simulink model "quadrotorVehicle_baseline_workshop"  (R2023b)
settings: Solver=VariableStepAuto  StartTime=0.0  StopTime=600  MaxStep=0.1  RelTol=1e-3  EnableMultiTasking=on
InitFcn:
  | % load parameters of the default quadrotor
  | disp('Quadrotor parameters loaded by InitFcn')
  | mdl_quadrotor;
  | waypoints = randi([-500,500],10,2);
libraries: simulink x2, slpidlib x1, roblocks x1
settings Model: PacingRate=10  Creator=corkep  LastModifiedBy=mejiasal
settings SolverCC: AlgebraicLoopSolver=TrustRegion
settings DataIOCC: LimitDataPoints=on  SaveFormat=Array  ReturnWorkspaceOutputs=off
settings OptimizationCC: BlockReduction=off  BooleanDataType=off  ReuseModelBlockBuffer=off  LifeSpan=inf
settings DebuggingCC: SaveWithParameterizedLinksMsg=none  MergeDetectMultiDrivingBlocksExec=none  SignalResolutionControl=TryResolveAllWithWarning  UnconnectedInputMsg=warning  UnconnectedOutputMsg=warning  UnconnectedLineMsg=warning  SFUnexpectedBacktrackingDiag=warning  SFNoUnconditionalDefaultTransitionDiag=warning  SFExecutionAtInitializationDiag=none  ArithmeticOperatorsInVariantConditions=warning
settings HardwareCC: ProdBitPerPointer=32  ProdBitPerSizeT=32  ProdBitPerPtrDiffT=32  ProdLargestAtomicFloat=None  ProdIntDivRoundTo=Undefined  ProdEndianess=Unspecified  ProdWordSize=32  ProdHWDeviceType=32-bit Generic  TargetUnknown=on
settings ModelReferenceCC: EnableRefExpFcnMdlSchedulingChecks=on  PropagateSignalLabelsOutOfModel=off
settings SFSimCC: SimUseLocalCustomCode=off  CustomCodeUndefinedFunction=UseInterfaceOnly
settings RTWCC: RTWUseLocalCustomCode=off
settings CodeAppCC: StateflowObjectComments=on
settings GRTTargetCC: TargetLangStandard=C89/C90 (ANSI)
settings ConfigComp: CovMetricSettings=dw  CovSaveCumulativeToWorkspaceVar=on  CovSaveSingleToWorkspaceVar=on  CovExternalEMLEnable=off  CovSFcnEnable=off

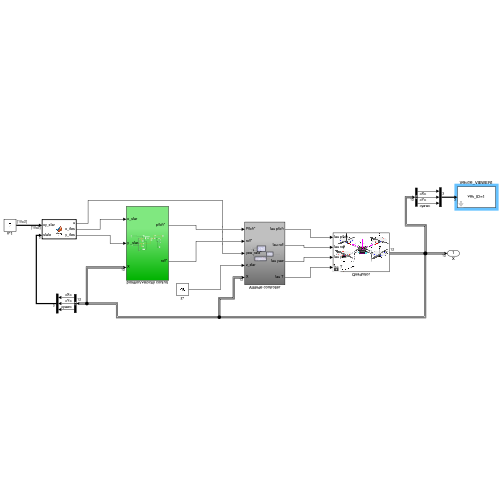
[thumbnail: Simulink's stored preview of the top-level diagram]
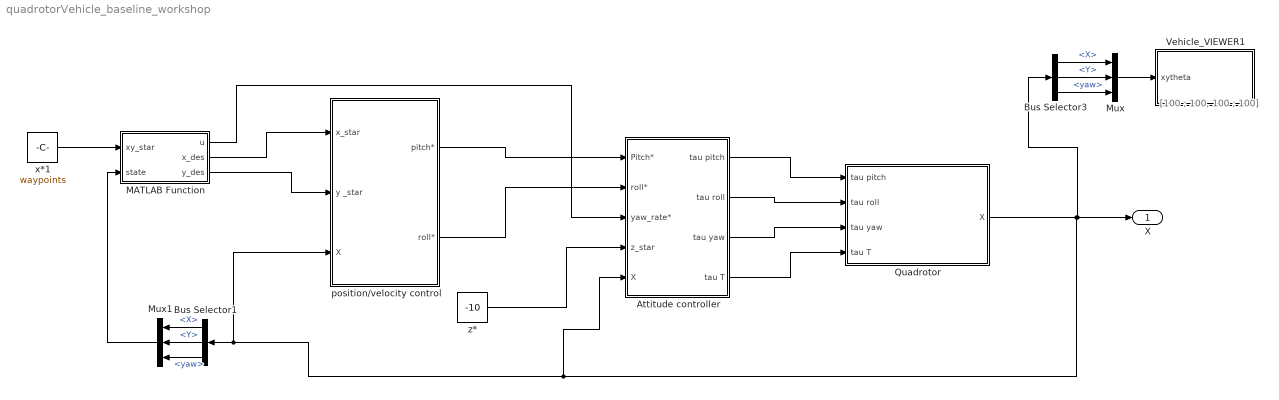
== system quadrotorVehicle_baseline_workshop ==
  note: [100 ; 100, 100 ; 100]
  Attitude controller : Subsystem
  Bus Selector1 : BusSelector  OutputSignals=X,Y,yaw
  Bus Selector3 : BusSelector  OutputSignals=X,Y,yaw
  MATLAB Function : MATLAB Function  TreatAsAtomicUnit=on
  Mux : Mux  Inputs=3
  Mux1 : Mux  Inputs=3
  Quadrotor : Subsystem
      mask Display: image('quadrotor.png');
  Vehicle_VIEWER1 : Subsystem  mask{wp_mat=waypoints, veh_ID_num=1, veh_init_xytheta=[0 0 0], Ts=5}
      mask prompts: wp_mat "Waypoint matrix for arena [x_col, y_col, z_col, angle_col] (m, deg)"; veh_ID_num "Vehicle ID number"; veh_init_xytheta "Initial pose [x,y, psi]"; Ts "Sample time for updating animation (secs)"
      mask TypeOptions veh_ID_num: 1 | 2 | 3 | 4
      mask DialogControl Control2 Prompt: Animate simulation of Robot
      mask Display: fprintf('veh_ID=%d',veh_ID_num);
  position/velocity control : Subsystem
  x*1 : Constant  Value=waypoints
  z* : Constant  Value=-10
  X : Outport
  wires:
  Bus Selector3/1 -> Mux/1  "<X>"
  Bus Selector3/2 -> Mux/2  "<Y>"
  Bus Selector3/3 -> Mux/3  "<yaw>"
  Mux/1 -> Vehicle_VIEWER1/1(xytheta)
  position/velocity control/2(roll*) -> Attitude controller/2(roll*)
  z*/1 -> Attitude controller/4(z_star)
  position/velocity control/1("pitch*  ") -> Attitude controller/1(Pitch*)
  Attitude controller/1(tau pitch) -> Quadrotor/1(tau pitch)
  Attitude controller/2(tau roll) -> Quadrotor/2(tau roll)
  Attitude controller/3(tau yaw) -> Quadrotor/3(tau yaw)
  Attitude controller/4(tau T) -> Quadrotor/4(tau T)
  Quadrotor/1(X) -> Bus Selector3/1, X/1, Attitude controller/5(X), position/velocity control/3(X), Bus Selector1/1
  Bus Selector1/1 -> Mux1/1  "<X>"
  Bus Selector1/2 -> Mux1/2  "<Y>"
  Bus Selector1/3 -> Mux1/3  "<yaw>"
  Mux1/1 -> MATLAB Function/2(state)
  MATLAB Function/1(u) -> Attitude controller/3(yaw_rate*)
  MATLAB Function/2(x_des) -> position/velocity control/1(x_star)
  MATLAB Function/3(y_des) -> position/velocity control/2(y _star)
  x*1/1 -> MATLAB Function/1(xy_star)

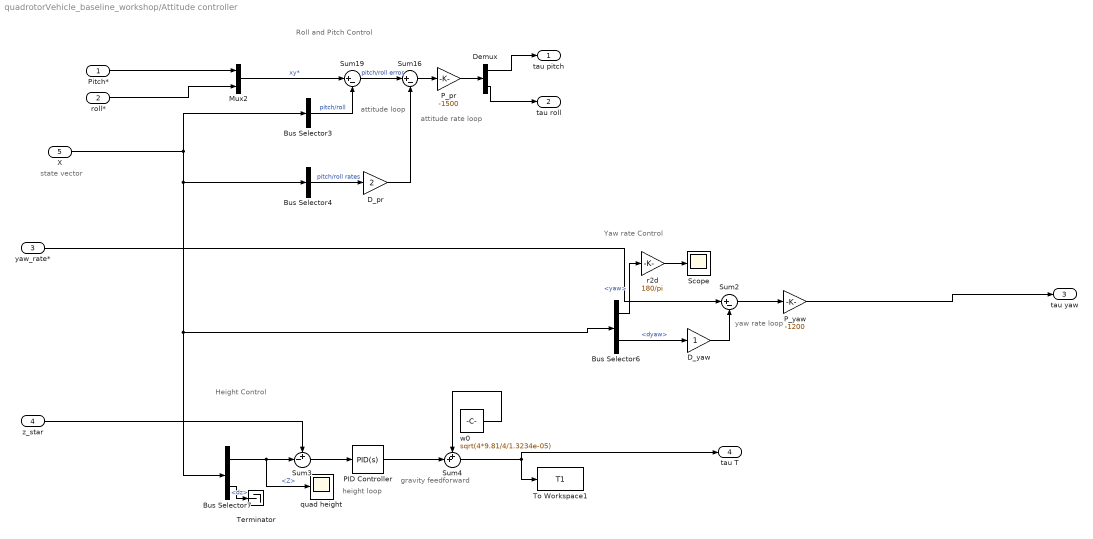
== system quadrotorVehicle_baseline_workshop/Attitude controller ==
  note: Height Control
  note: Yaw rate Control
  note: Roll and Pitch Control
  note: state vector
  note: gravity feedforward
  note: attitude rate
      | loop
  note: height
      | loop
  note: attitude
      | loop
  note: yaw rate
      | loop
  Pitch* : Inport
  roll* : Inport  Port=2
  yaw_rate* : Inport  Port=3
  z_star : Inport  Port=4
  X : Inport  Port=5
  Bus Selector3 : BusSelector  OutputSignals=pitch,roll  OutputAsBus=on
  Bus Selector4 : BusSelector  OutputSignals=dpitch,droll  OutputAsBus=on
  Bus Selector6 : BusSelector  OutputSignals=yaw,dyaw
  Bus Selector7 : BusSelector  OutputSignals=Z,dz
  D_pr : Gain  Gain=2
  D_yaw : Gain
  Demux : Demux  Outputs=2
  Mux2 : Mux  Inputs=2
  PID Controller : slpidlib/PID Controller  Controller=PID  Form=Parallel  TimeDomain=Continuous-time  UseExternalTs=off  SampleTime=-1  IntegratorMethod=Forward Euler  FilterMethod=Forward Euler  ControllerParametersSource=internal  P=-7.01788852939257  I=-0.1  UseKiTs=off  D=-38  N=5.45397025421619  UseFilter=on  TunerSelectOption=Transfer Function Based (PID Tuner App)  InitialConditionSource=internal  InitialConditionForIntegrator=0  InitialConditionForFilter=0  DifferentiatorICPrevScaledInput=0  ExternalReset=none  TrackingMode=off  Kt=1  LimitOutput=off  SatLimitsSource=internal  UpperSaturationLimit=inf  LowerSaturationLimit=-inf  LinearizeAsGain=on  AntiWindupMode=none  Kb=1  LimitIntegrator=off  UpperIntegratorSaturationLimit=inf  LowerIntegratorSaturationLimit=-inf  POutMin=[]  POutMax=[]  IOutMin=[]  IOutMax=[]  DOutMin=[]  DOutMax=[]  NOutMin=[]  NOutMax=[]  SumOutMin=[]  SumOutMax=[]  SaturationOutMin=[]  SaturationOutMax=[]  PParamMin=[]  PParamMax=[]  IParamMin=[]  IParamMax=[]  DParamMin=[]  DParamMax=[]  NParamMin=[]  NParamMax=[]  KbParamMin=[]  KbParamMax=[]  KtParamMin=[]  KtParamMax=[]  KbOutMin=[]  KbOutMax=[]  KtOutMin=[]  KtOutMax=[]  IntegratorOutMin=[]  IntegratorOutMax=[]  FilterOutMin=[]  FilterOutMax=[]  SumI1OutMin=[]  SumI1OutMax=[]  SumI2OutMin=[]  SumI2OutMax=[]  SumI3OutMin=[]  SumI3OutMax=[]  SumI4OutMin=[]  SumI4OutMax=[]  SumDOutMin=[]  SumDOutMax=[]  DifferentiatorOutMin=[]  DifferentiatorOutMax=[]  FilterDiffOutCoefMin=[]  FilterDiffOutCoefMax=[]  ReciprocalOutMin=[]  ReciprocalOutMax=[]  SumDenOutMin=[]  SumDenOutMax=[]  SumNumOutMin=[]  SumNumOutMax=[]  DivideOutMin=[]  DivideOutMax=[]  UdiffTsProdOutMin=[]  UdiffTsProdOutMax=[]  NTsProdOutMin=[]  NTsProdOutMax=[]  UintegralTsProdOutMin=[]  UintegralTsProdOutMax=[]  UngainTsProdOutMin=[]  UngainTsProdOutMax=[]  ClampingZeroOutDataTypeStr=Inherit: Inherit via back propagation  ClampingZeroOutMin=[]  ClampingZeroOutMax=[]  FilterDenConstantOutDataTypeStr=Inherit: Inherit via back propagation  FilterDenConstantOutMin=[]  FilterDenConstantOutMax=[]  PCopyOutDataTypeStr=Inherit: Inherit via back propagation  PCopyOutMin=[]  PCopyOutMax=[]  NCopyOutDataTypeStr=Inherit: Inherit via back propagation  NCopyOutMin=[]  NCopyOutMax=[]  IntegratorContinuousStateAttributes=''  IntegratorStateMustResolveToSignalObject=off  IntegratorRTWStateStorageClass=Auto  FilterContinuousStateAttributes=''  FilterStateMustResolveToSignalObject=off  FilterRTWStateStorageClass=Auto  ParallelPVariant=InternalParameters  IdealPVariant=Disabled  IVariant=InternalParameters  DVariant=InternalParameters  IntegratorVariant=Continuous  SatVariant=Disabled  AWVariant=Passthrough  PCopyVariant=Disabled  TRVariant=Disabled  FdbkBlocksVariant=Forward  IdealPFdbkVariant=Disabled  SatFdbkVariant=Disabled  DerivativeFilterVariant=ContFilter  NVariant=InternalParameters  NCopyVariant=Disabled  FilterICVariant=InternalICsFilter  IntegratorICVariant=InternalICs  ExternalResetVariant=Disabled  TRSumVariant=Passthrough  SumFdbkVariant=Disabled  SumVariant=Sum_PID  TsampFilterVariant=InternalTs  TsampNgainVariant=Passthrough  TsampIntegralVariant=Disabled_SignalSpec  ExternalSaturationOutDataTypeStr=Inherit: Same as second input
  P_pr : Gain  Gain=-1500
  P_yaw : Gain  Gain=-1200
  Scope : Scope
  Sum16 : Sum  Inputs=|+-
  Sum19 : Sum  Inputs=|+-
  Sum2 : Sum  Inputs=|+-
  Sum3 : Sum  Inputs=+-|
  Sum4 : Sum  Inputs=++|
  Terminator : Terminator
  To Workspace1 : ToWorkspace  VariableName=T1  SampleTime=-1
  quad height : Scope
  r2d : Gain  Gain=180/pi
  w0 : Constant  Value=sqrt(4*9.81/4/1.3234e-05)  SampleTime=0
  tau pitch : Outport  VectorParamsAs1DForOutWhenUnconnected=off
  tau roll : Outport  Port=2  VectorParamsAs1DForOutWhenUnconnected=off
  tau yaw : Outport  Port=3  VectorParamsAs1DForOutWhenUnconnected=off
  tau T : Outport  Port=4  VectorParamsAs1DForOutWhenUnconnected=off
  wires:
  P_pr/1 -> Demux/1
  Demux/1 -> tau pitch/1
  yaw_rate*/1 -> Sum2/1
  roll*/1 -> Mux2/2
  Bus Selector6/1 -> r2d/1  "<yaw>"
  Bus Selector3/1 -> Sum19/2  "pitch/roll"
  PID Controller/1 -> Sum4/2
  Demux/2 -> tau roll/1
  Sum16/1 -> P_pr/1
  Mux2/1 -> Sum19/1  "xy*"
  r2d/1 -> Scope/1
  z_star/1 -> Sum3/1
  Sum19/1 -> Sum16/1  "pitch/roll error"
  Pitch*/1 -> Mux2/1
  D_yaw/1 -> Sum2/2
  Bus Selector6/2 -> D_yaw/1  "<dyaw>"
  Bus Selector4/1 -> D_pr/1  "pitch/roll rates"
  Bus Selector7/1 -> quad height/1, Sum3/2  "<Z>"
  X/1 -> Bus Selector7/1, Bus Selector6/1, Bus Selector4/1, Bus Selector3/1
  Sum2/1 -> P_yaw/1
  Sum3/1 -> PID Controller/1
  w0/1 -> Sum4/1
  D_pr/1 -> Sum16/2
  P_yaw/1 -> tau yaw/1
  Sum4/1 -> tau T/1, To Workspace1/1
  Bus Selector7/2 -> Terminator/1  "<dz>"

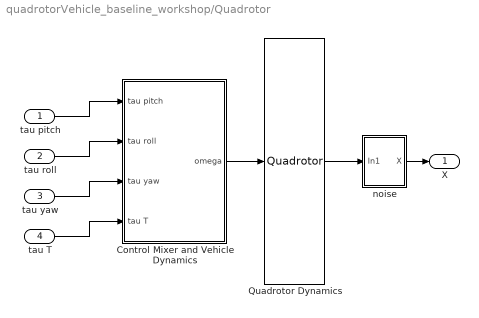
== system quadrotorVehicle_baseline_workshop/Quadrotor ==
  tau pitch : Inport
  tau roll : Inport  Port=2
  tau yaw : Inport  Port=3
  tau T : Inport  Port=4
  Control Mixer and Vehicle Dynamics : Subsystem
  Quadrotor Dynamics : roblocks/Dynamics/Quadrotor  quad=quad
  noise : Subsystem
  X : Outport
  wires:
  tau yaw/1 -> Control Mixer and Vehicle Dynamics/3(tau yaw)
  tau T/1 -> Control Mixer and Vehicle Dynamics/4(tau T)
  Control Mixer and Vehicle Dynamics/1(omega) -> Quadrotor Dynamics/1
  tau roll/1 -> Control Mixer and Vehicle Dynamics/2(tau roll)
  tau pitch/1 -> Control Mixer and Vehicle Dynamics/1(tau pitch)
  Quadrotor Dynamics/1 -> noise/1(In1)
  noise/1(X) -> X/1

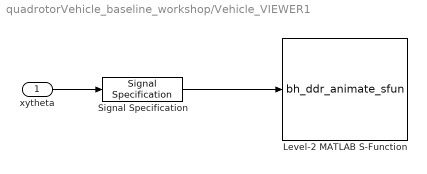
== system quadrotorVehicle_baseline_workshop/Vehicle_VIEWER1 ==
  xytheta : Inport
  Level-2 MATLAB S-Function : M-S-Function  FunctionName=bh_ddr_animate_sfun  Parameters=Ts, wp_mat, veh_ID_num, veh_init_xytheta
  Signal Specification : SignalSpecification  Dimensions=3
  wires:
  xytheta/1 -> Signal Specification/1
  Signal Specification/1 -> Level-2 MATLAB S-Function/1

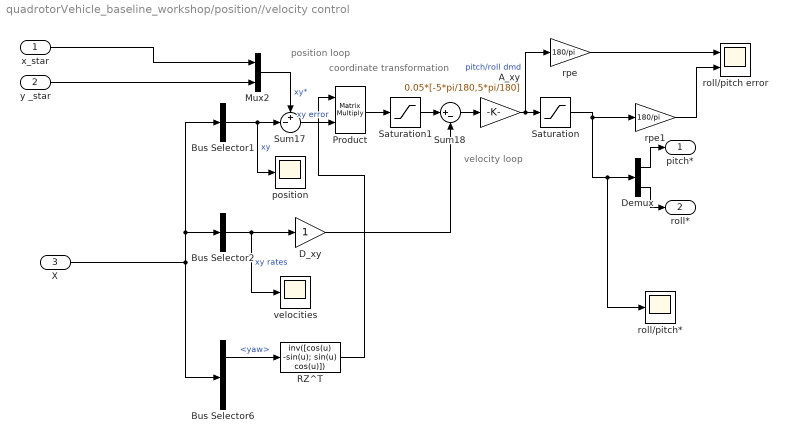
== system quadrotorVehicle_baseline_workshop/position//velocity control ==
  note: position
      | loop
  note: velocity
      | loop
  note: coordinate transformation
  x_star : Inport
  y _star : Inport  Port=2
  X : Inport  Port=3
  A_xy : Gain  Gain=0.05*[-5*pi/180,5*pi/180]
  Bus Selector1 : BusSelector  OutputSignals=X,Y  OutputAsBus=on
  Bus Selector2 : BusSelector  OutputSignals=dx,dy  OutputAsBus=on
  Bus Selector6 : BusSelector  OutputSignals=yaw,dyaw
  D_xy : Gain
  Demux : Demux  Outputs=2
  Mux2 : Mux  Inputs=2
  Product : Product  Multiplication=Matrix(*)  RndMeth=Zero
  RZ^T : MATLABFcn  MATLABFcn=inv([cos(u) -sin(u); sin(u) cos(u)])  OutputDimensions=[2 2]  Output1D=off
  Saturation : Saturate  UpperLimit=5*pi/180  LowerLimit=-5*pi/180
  Saturation1 : Saturate  UpperLimit=5  LowerLimit=-5
  Sum17 : Sum  Inputs=+-|
  Sum18 : Sum  Inputs=|+-
  position : Scope
  roll/pitch error : Scope  NumInputPorts=2
  roll/pitch* : Scope
  rpe : Gain  Gain=180/pi
  rpe1 : Gain  Gain=180/pi
  velocities : Scope
  "pitch*  " : Outport  VectorParamsAs1DForOutWhenUnconnected=off
  roll* : Outport  Port=2  VectorParamsAs1DForOutWhenUnconnected=off
  wires:
  Demux/2 -> roll*/1
  Demux/1 -> "pitch*  "/1
  Product/1 -> Saturation1/1
  D_xy/1 -> Sum18/2
  Sum18/1 -> A_xy/1
  Bus Selector6/1 -> RZ^T/1  "<yaw>"
  Sum17/1 -> Product/2  "xy error"
  Mux2/1 -> Sum17/1  "xy*"
  Bus Selector2/1 -> velocities/1, D_xy/1  "xy rates"
  RZ^T/1 -> Product/1
  Saturation/1 -> rpe1/1, roll/pitch*/1, Demux/1
  X/1 -> Bus Selector1/1, Bus Selector2/1, Bus Selector6/1
  Bus Selector1/1 -> position/1, Sum17/2  "xy"
  x_star/1 -> Mux2/1
  y _star/1 -> Mux2/2
  A_xy/1 -> rpe/1, Saturation/1  "pitch/roll dmd"
  rpe/1 -> roll/pitch error/1
  rpe1/1 -> roll/pitch error/2
  Saturation1/1 -> Sum18/1

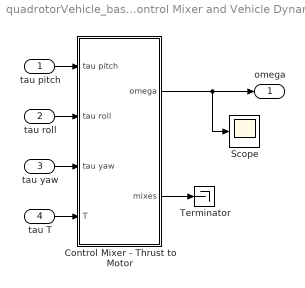
== system quadrotorVehicle_baseline_workshop/Quadrotor/Control Mixer and Vehicle Dynamics ==
  tau pitch : Inport
  tau roll : Inport  Port=2
  tau yaw : Inport  Port=3
  tau T : Inport  Port=4
  Control Mixer - Thrust to Motor : Subsystem
  Scope : Scope
  Terminator : Terminator
  omega : Outport  VectorParamsAs1DForOutWhenUnconnected=off
  wires:
  Control Mixer - Thrust to Motor/2(mixes) -> Terminator/1
  tau pitch/1 -> Control Mixer - Thrust to Motor/1(tau pitch)
  tau roll/1 -> Control Mixer - Thrust to Motor/2(tau roll)
  tau yaw/1 -> Control Mixer - Thrust to Motor/3(tau yaw)
  tau T/1 -> Control Mixer - Thrust to Motor/4(T)
  Control Mixer - Thrust to Motor/1(omega) -> Scope/1, omega/1

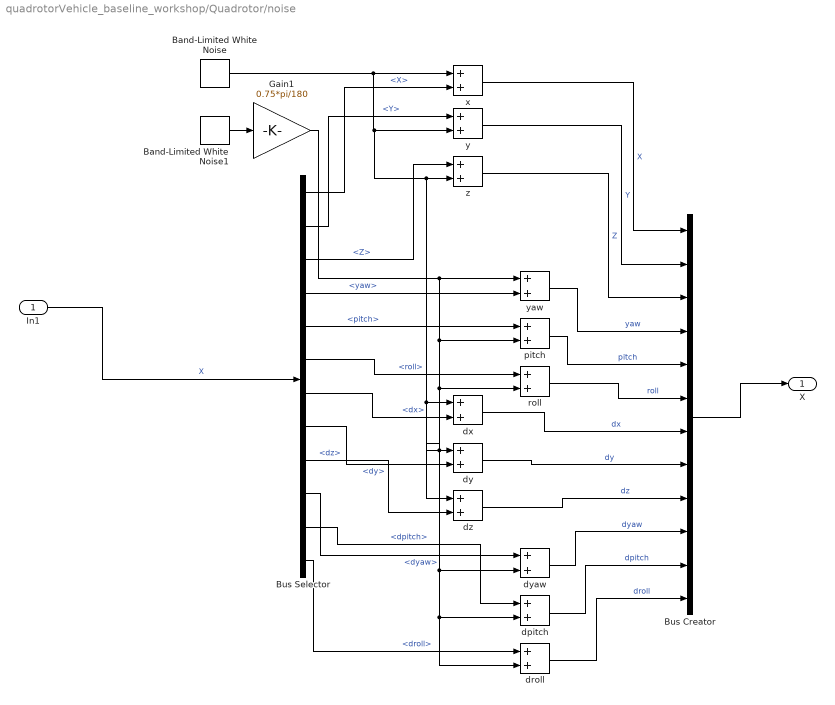
== system quadrotorVehicle_baseline_workshop/Quadrotor/noise ==
  In1 : Inport
  Band-Limited White Noise : simulink/Sources/Band-Limited White Noise  Cov=[0.001]  Ts=0.1  seed=[23341]
  Band-Limited White Noise1 : simulink/Sources/Band-Limited White Noise  Cov=[0.41]  Ts=0.1  seed=[23341]
  Bus Creator : BusCreator  Inputs=12
  Bus Selector : BusSelector  OutputSignals=X,Y,Z,yaw,pitch,roll,dx,dy,dz,dyaw,dpitch,droll
  Gain1 : Gain  Gain=0.75*pi/180
  dpitch : Sum
  droll : Sum
  dx : Sum
  dy : Sum
  dyaw : Sum
  dz : Sum
  pitch : Sum
  roll : Sum
  x : Sum
  y : Sum
  yaw : Sum
  z : Sum
  X : Outport
  wires:
  x/1 -> Bus Creator/1  "X"
  Bus Selector/9 -> dz/2  "<dz>"
  Bus Selector/8 -> dy/2  "<dy>"
  Bus Selector/7 -> dx/2  "<dx>"
  y/1 -> Bus Creator/2  "Y"
  Bus Selector/6 -> roll/1  "<roll>"
  Bus Selector/5 -> pitch/1  "<pitch>"
  yaw/1 -> Bus Creator/4  "yaw"
  Bus Selector/2 -> y/1  "<Y>"
  Bus Selector/1 -> x/2  "<X>"
  Gain1/1 -> pitch/2, droll/2, dpitch/2, dyaw/2, roll/2, yaw/1
  Band-Limited White Noise/1 -> x/1, z/2, dx/1, dz/1, dy/1, y/2
  Bus Selector/10 -> dyaw/1  "<dyaw>"
  Bus Selector/11 -> dpitch/1  "<dpitch>"
  Bus Selector/4 -> yaw/2  "<yaw>"
  Bus Selector/12 -> droll/1  "<droll>"
  Band-Limited White Noise1/1 -> Gain1/1
  Bus Selector/3 -> z/1  "<Z>"
  z/1 -> Bus Creator/3  "Z"
  In1/1 -> Bus Selector/1  "X"
  Bus Creator/1 -> X/1
  pitch/1 -> Bus Creator/5  "pitch"
  roll/1 -> Bus Creator/6  "roll"
  dpitch/1 -> Bus Creator/11  "dpitch"
  droll/1 -> Bus Creator/12  "droll"
  dx/1 -> Bus Creator/7  "dx"
  dy/1 -> Bus Creator/8  "dy"
  dz/1 -> Bus Creator/9  "dz"
  dyaw/1 -> Bus Creator/10  "dyaw"

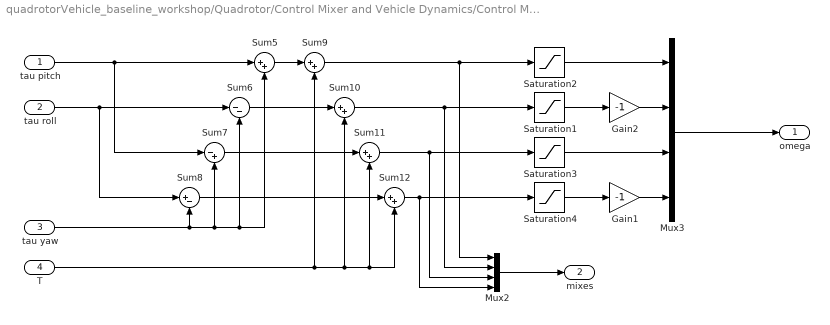
== system quadrotorVehicle_baseline_workshop/Quadrotor/Control Mixer and Vehicle Dynamics/Control Mixer - Thrust to Motor ==
  tau pitch : Inport
  tau roll : Inport  Port=2
  tau yaw : Inport  Port=3
  T : Inport  Port=4
  Gain1 : Gain  Gain=-1
  Gain2 : Gain  Gain=-1
  Mux2 : Mux
  Mux3 : Mux
  Saturation{1..4} (4 alike) : Saturate  UpperLimit=1000  LowerLimit=700
  Sum{5,9..12} (5 alike) : Sum  Inputs=|++  InputSameDT=on  SaturateOnIntegerOverflow=on  OutDataTypeStr=Inherit: Same as first input
  Sum6 : Sum  Inputs=|--  InputSameDT=on  SaturateOnIntegerOverflow=on  OutDataTypeStr=Inherit: Same as first input
  Sum7 : Sum  Inputs=|-+  InputSameDT=on  SaturateOnIntegerOverflow=on  OutDataTypeStr=Inherit: Same as first input
  Sum8 : Sum  Inputs=|+-  InputSameDT=on  SaturateOnIntegerOverflow=on  OutDataTypeStr=Inherit: Same as first input
  omega : Outport  VectorParamsAs1DForOutWhenUnconnected=off
  mixes : Outport  Port=2  VectorParamsAs1DForOutWhenUnconnected=off
  wires:
  Sum7/1 -> Sum11/1
  tau roll/1 -> Sum6/1, Sum8/1
  Mux2/1 -> mixes/1
  Gain2/1 -> Mux3/2
  Sum8/1 -> Sum12/1
  Sum6/1 -> Sum10/1
  tau pitch/1 -> Sum5/1, Sum7/1
  Mux3/1 -> omega/1
  Sum10/1 -> Saturation1/1, Mux2/2
  Sum12/1 -> Saturation4/1, Mux2/4
  Saturation1/1 -> Gain2/1
  Saturation3/1 -> Mux3/3
  T/1 -> Sum11/2, Sum12/2, Sum10/2, Sum9/2
  tau yaw/1 -> Sum8/2, Sum7/2, Sum6/2, Sum5/2
  Saturation4/1 -> Gain1/1
  Sum9/1 -> Saturation2/1, Mux2/1
  Sum11/1 -> Saturation3/1, Mux2/3
  Saturation2/1 -> Mux3/1
  Sum5/1 -> Sum9/1
  Gain1/1 -> Mux3/4

== matlab function quadrotorVehicle_baseline_workshop/MATLAB Function ==
  settings: updateMethod=DISCRETE
  data: xy_star input; u output; state input; x_des output; y_des output
function [u, x_des, y_des] = fcn(xy_star, state)

persistent index;

if isempty(index)
    index=1;
end


u = 0.0;
k = 0.73;
e = 0.0;
x_des=0.0;
y_des=0.0;



len = length(xy_star);

x_star=xy_star(:,1);
y_star=xy_star(:,2);

xd=x_star(index);
yd=y_star(index);

x_des = xd;
y_des = yd;


x=state(1);
y=state(2);
theta=state(3);

%use distance to current waypoint
d = sqrt((xd-x)^2 + (yd-y)^2)

theta_star = atan2(yd-y,xd-x);

%e = theta_star - theta
e = angdiff(theta,theta_star);

u =  k * e; % k* ( theta_star - theta)

if d < 5
    index = index+1;
else
    index = index;
end

 if index > len
     index = 1;
 end

end
